simulink model "Ex2_Motor_Model"  (R2025b)
settings: Solver=ode45  StartTime=0.0  StopTime=2  RelTol=1e-3
PreLoadFcn:
  | Kp=0;
  | Ki=0;
  | Kd=0
InitFcn:
  | J = 0.01;
  | b = 0.1;
  | K = 0.01;
  | R = 1;
  | L = 0.5;
settings Model: Creator=sansh  LastModifiedBy=sjawahar
settings SolverCC: AlgebraicLoopSolver=TrustRegion
settings DataIOCC: ReturnWorkspaceOutputs=off
settings DebuggingCC: UnconnectedInputMsg=warning  UnconnectedOutputMsg=warning  UnconnectedLineMsg=warning  ArithmeticOperatorsInVariantConditions=warning
settings ModelReferenceCC: EnableRefExpFcnMdlSchedulingChecks=on
settings SFSimCC: SimUseLocalCustomCode=off  CustomCodeUndefinedFunction=UseInterfaceOnly
settings RTWCC: RTWUseLocalCustomCode=off  GPUComputeCapability=3.5
settings CodeAppCC: StateflowObjectComments=on

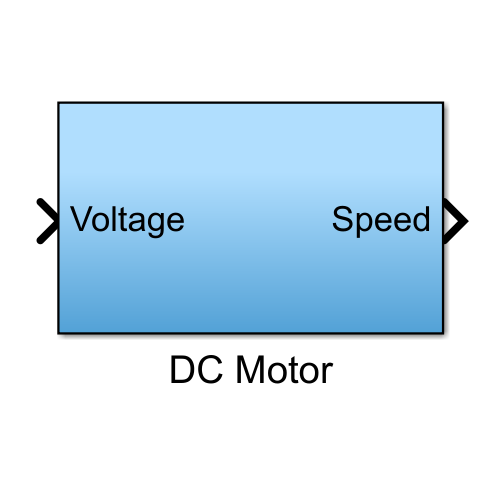
[thumbnail: Simulink's stored preview of the top-level diagram]
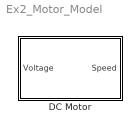
== system Ex2_Motor_Model ==
  DC Motor : Subsystem

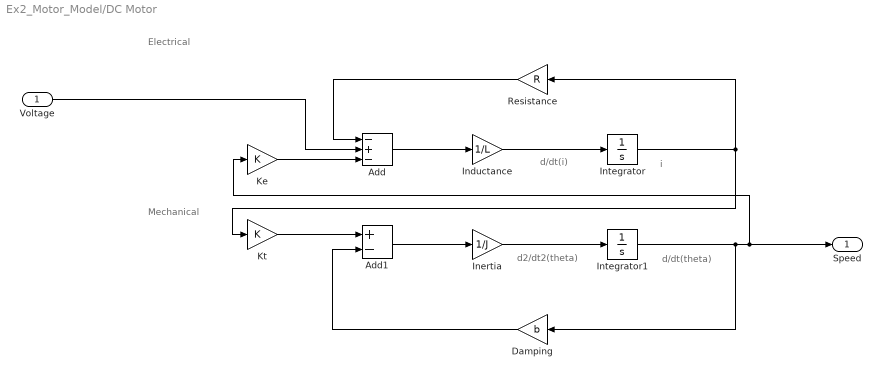
== system Ex2_Motor_Model/DC Motor ==
  note: Electrical
  note: Mechanical
  note: i
  note: d/dt(i)
  note: d/dt(theta)
  note: d2/dt2(theta)
  Voltage : Inport
  Add : Sum  Inputs=-+-
  Add1 : Sum  Inputs=+-
  Damping : Gain  Gain=b
  Inductance : Gain  Gain=1/L
  Inertia : Gain  Gain=1/J
  Integrator : Integrator
  Integrator1 : Integrator
  Ke : Gain  Gain=K
  Kt : Gain  Gain=K
  Resistance : Gain  Gain=R
  Speed : Outport
  wires:
  Inductance/1 -> Integrator/1
  Integrator1/1 -> Damping/1, Speed/1, Ke/1
  Inertia/1 -> Integrator1/1
  Integrator/1 -> Resistance/1, Kt/1
  Kt/1 -> Add1/1
  Voltage/1 -> Add/2
  Resistance/1 -> Add/1
  Damping/1 -> Add1/2
  Ke/1 -> Add/3
  Add/1 -> Inductance/1
  Add1/1 -> Inertia/1
